simulink model "autoquet_simulink"  (R2023b)
settings: Solver=FixedStepAuto  StartTime=0.0  StopTime=600  FixedStep=1e-3  RelTol=1e-3
libraries: arduinolib x8, dspfdesign x2, arduinosensorlib x1
settings Model: ExtModeTrigDuration=2  Creator=doria  LastModifiedBy=doria
settings OptimizationCC: EnhancedBackFolding=on  PassReuseOutputArgsAs=Individual arguments  ZeroExternalMemoryAtStartup=off  ZeroInternalMemoryAtStartup=off  MaxStackSize=64  OptimizeBlockOrder=speed  DifferentSizesBufferReuse=on  OptimizationCustomize=off  EfficientTunableParamExpr=on
settings DebuggingCC: ParameterTunabilityLossMsg=error
settings HardwareCC: ProdBitPerInt=16  ProdBitPerPointer=16  ProdBitPerSizeT=16  ProdBitPerPtrDiffT=16  ProdLargestAtomicFloat=None  ProdWordSize=8  ProdHWDeviceType=Atmel->AVR
settings SFSimCC: MATLABDynamicMemAlloc=off
settings RTWCC: Description=Embedded Coder  SystemTargetFile=ert.tlc  HardwareBoard=Arduino Leonardo  TemplateMakefile=ert_default_tmf  Toolchain=Arduino AVR  BuildConfiguration=Faster Runs
settings CodeAppCC: ForceParamTrailComments=on  IgnoreCustomStorageClasses=off  OperatorAnnotations=on  SimulinkDataObjDesc=on  SFDataObjDesc=on  InsertBlockDesc=on
settings ERTTargetCC: SupportContinuousTime=on  SupportVariableSizeSignals=on  ExtModeTransport=3  ExtModeStaticAlloc=on  ExtModeAutomaticAllocSize=off  ExtModeStaticAllocSize=250  ExtModeMexFile=ext_xcp  ExtModeIntrfLevel=Level2 - Open

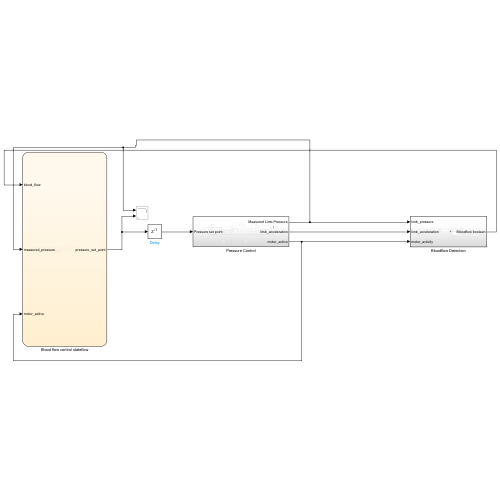
[thumbnail: Simulink's stored preview of the top-level diagram]
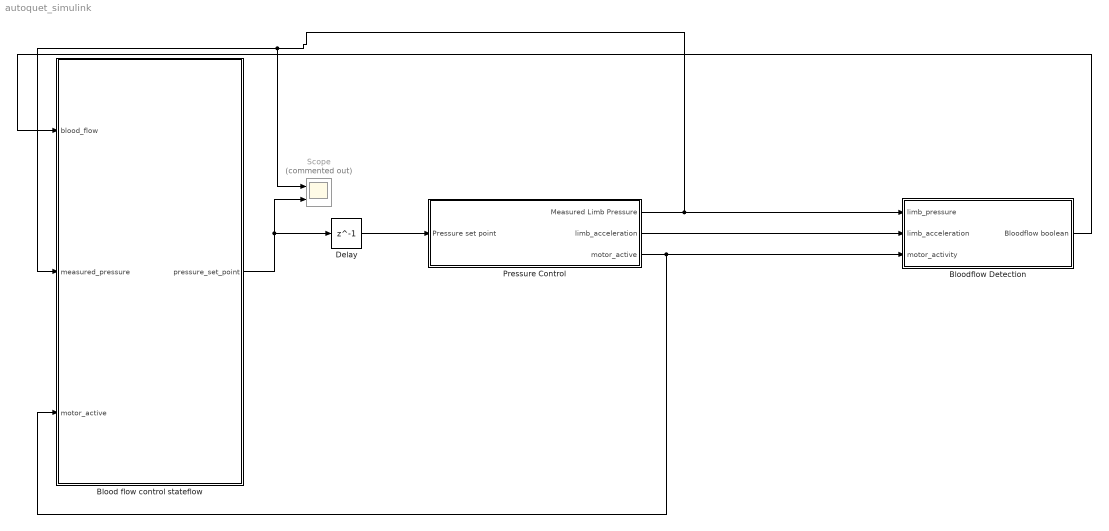
== system autoquet_simulink ==
  Blood flow control stateflow : Stateflow chart  TreatAsAtomicUnit=on
  Bloodflow Detection : Subsystem
  Delay : Delay  DelayLength=1  InitialCondition=100
  Pressure Control : Subsystem
  Scope : Scope  Commented=on  NumInputPorts=2
  wires:
  Delay/1 -> Pressure Control/1(Pressure set point)
  Pressure Control/1(Measured Limb Pressure) -> Bloodflow Detection/1(limb_pressure), Blood flow control stateflow/2(measured_pressure), Scope/1
  Bloodflow Detection/1(Bloodflow boolean) -> Blood flow control stateflow/1(blood_flow)
  Pressure Control/3(motor_active) -> Blood flow control stateflow/3(motor_active), Bloodflow Detection/3(motor_activity)
  Blood flow control stateflow/1(pressure_set_point) -> Delay/1, Scope/2
  Pressure Control/2(limb_acceleration) -> Bloodflow Detection/2(limb_acceleration)

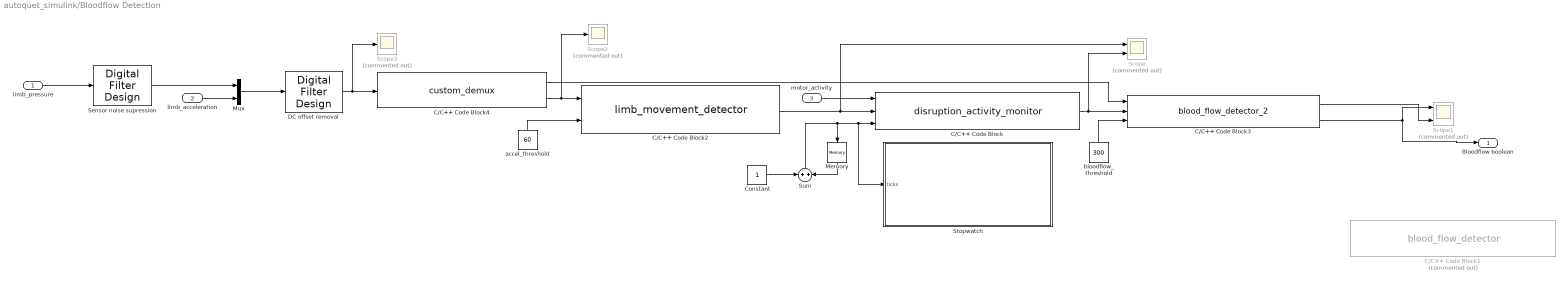
== system autoquet_simulink/Bloodflow Detection ==
  limb_pressure : Inport
  limb_acceleration : Inport  Port=2
  motor_activity : Inport  Port=3
  C/C++ Code Block : S-Function  FunctionName=disruption_activity_monitor  SFunctionModules=disruption_activity_monitor_wrapper.c  SFunctionDeploymentMode=off  EnableBusSupport=off  mask(S-Function Builder){}
      mask help: Simulink:masks:SFunctionBuilder_MD
      mask init:
      | val = [[.9  0.75 0.75 1 1 .9 .9 1]',[1 1 0.75 0.75 .9 .9 1 .9]'];try , sys = get_param(gcb,'SfunBuilderFcnName');if isempty(sys), sys = get_param(gcb,'FunctionName'); end,catch, sys = get_param(gcb,'FunctionName'); end
      settings: CopyFcn=set_param(gcbh,'LinkStatus','none')  OpenFcn=sfunctionwizard(gcbh)
      mask Display:
      | plot(val(:,1),val(:,2))
      | disp(sys)
      | port_label('input',1,'motor_active')
      | port_label('input',2,'movement_detected')
      | port_label('input',3,'time')
      | port_label('output',1,'pause_summation')
  C/C++ Code Block1 : S-Function  Commented=on  FunctionName=blood_flow_detector  SFunctionModules=blood_flow_detector_wrapper.c  SFunctionDeploymentMode=off  EnableBusSupport=off  mask(S-Function Builder){}
      mask help: Simulink:masks:SFunctionBuilder_MD
      mask init: same as autoquet_simulink/Bloodflow Detection/C/C++ Code Block
      settings: CopyFcn=set_param(gcbh,'LinkStatus','none')  OpenFcn=sfunctionwizard(gcbh)
      mask Display: plot(val(:,1),val(:,2)),disp(sys),port_label('input',1,'u0'),port_label('input',2,'disruption_active'),port_label('input',3,'bloodflow_threshold'),port_label('output',1,'y0'),port_label('output',2,'bloodflow_boolean')
  C/C++ Code Block2 : S-Function  FunctionName=limb_movement_detector  SFunctionModules=limb_movement_detector_wrapper.c  SFunctionDeploymentMode=off  EnableBusSupport=off  mask(S-Function Builder){}
      mask help: Simulink:masks:SFunctionBuilder_MD
      mask init: same as autoquet_simulink/Bloodflow Detection/C/C++ Code Block
      settings: CopyFcn=set_param(gcbh,'LinkStatus','none')  OpenFcn=sfunctionwizard(gcbh)
      mask Display:
      | plot(val(:,1),val(:,2))
      | disp(sys)
      | port_label('input',1,'limb_acceleration')
      | port_label('input',2,'accel_threshold')
      | port_label('output',1,'movement_boolean')
  C/C++ Code Block3 : S-Function  FunctionName=blood_flow_detector_2  SFunctionModules=blood_flow_detector_2_wrapper.c  SFunctionDeploymentMode=off  EnableBusSupport=off  mask(S-Function Builder){}
      mask help: Simulink:masks:SFunctionBuilder_MD
      mask init: same as autoquet_simulink/Bloodflow Detection/C/C++ Code Block
      settings: CopyFcn=set_param(gcbh,'LinkStatus','none')  OpenFcn=sfunctionwizard(gcbh)
      mask Display:
      | plot(val(:,1),val(:,2))
      | disp(sys)
      | port_label('input',1,'u0')
      | port_label('input',2,'disruption_active')
      | port_label('input',3,'bloodflow_threshold')
      | port_label('output',1,'y0')
      | port_label('output',2,'bloodflow_boolean')
  C/C++ Code Block4 : S-Function  FunctionName=custom_demux  SFunctionModules=custom_demux_wrapper.c  SFunctionDeploymentMode=off  EnableBusSupport=off  mask(S-Function Builder){}
      mask help: Simulink:masks:SFunctionBuilder_MD
      mask init: same as autoquet_simulink/Bloodflow Detection/C/C++ Code Block
      settings: CopyFcn=set_param(gcbh,'LinkStatus','none')  OpenFcn=sfunctionwizard(gcbh)
      mask Display:
      | plot(val(:,1),val(:,2))
      | disp(sys)
      | port_label('input',1,'combined_vector')
      | port_label('output',1,'filtered_pressure')
      | port_label('output',2,'filtered_acceleration')
  Constant : Constant  OutDataTypeStr=uint32  SampleTime=0.1
  DC offset removal : dspfdesign/Digital Filter Design  mwdsp_browser_bugfix_var=off
  Memory : Memory
  Mux : Mux  Inputs=2
  Scope : Scope  Commented=on  NumInputPorts=2
  Scope1 : Scope  Commented=on  NumInputPorts=2
  Scope2 : Scope  Commented=on
  Scope3 : Scope  Commented=on
  Sensor noise supression : dspfdesign/Digital Filter Design  mwdsp_browser_bugfix_var=off
  Stopwatch : Subsystem
  Sum : Sum  Inputs=+|+
  accel_threshold : Constant  Value=60  OutDataTypeStr=uint16
  bloodflow_threshold : Constant  Value=300  OutDataTypeStr=uint16
  Bloodflow boolean : Outport
  wires:
  Mux/1 -> DC offset removal/1
  C/C++ Code Block/1 -> C/C++ Code Block3/2, Scope/2
  motor_activity/1 -> C/C++ Code Block/1
  C/C++ Code Block3/2 -> Bloodflow boolean/1, Scope1/1
  bloodflow_threshold/1 -> C/C++ Code Block3/3
  C/C++ Code Block3/1 -> Scope1/2
  Constant/1 -> Sum/1
  Memory/1 -> Sum/2
  accel_threshold/1 -> C/C++ Code Block2/2
  limb_pressure/1 -> Sensor noise supression/1
  Sensor noise supression/1 -> Mux/1
  DC offset removal/1 -> Scope3/1, C/C++ Code Block4/1
  C/C++ Code Block2/1 -> Scope/1, C/C++ Code Block/2
  Sum/1 -> Stopwatch/1(ticks), C/C++ Code Block/3, Memory/1
  limb_acceleration/1 -> Mux/2
  C/C++ Code Block4/1 -> C/C++ Code Block3/1
  C/C++ Code Block4/2 -> Scope2/1, C/C++ Code Block2/1

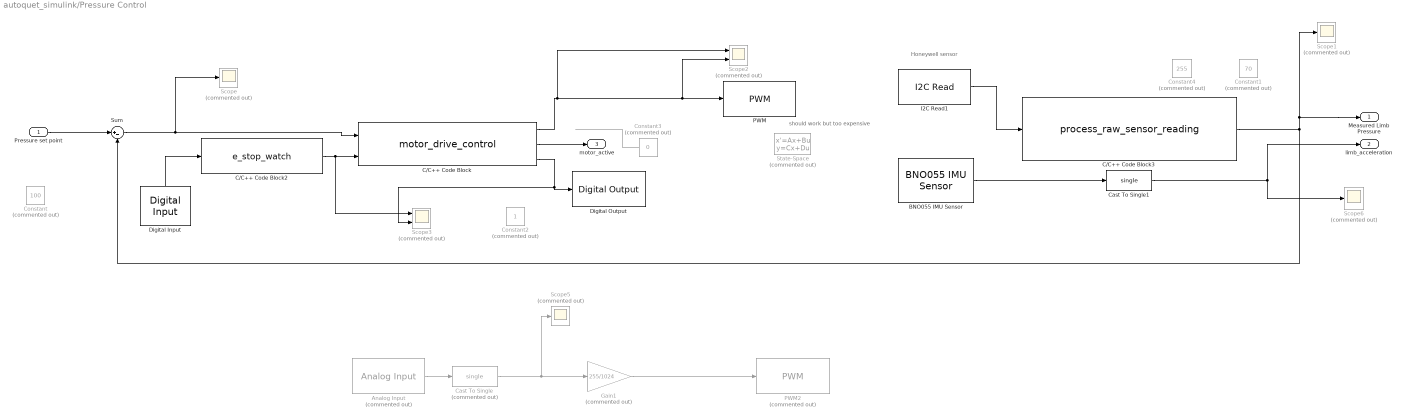
== system autoquet_simulink/Pressure Control ==
  note: should work but too expensive
  note: Honeywell sensor
  Pressure set point : Inport
  Analog Input : arduinolib/Analog Input  Commented=on  pinNumber=0  ReadResultsOnly=off  ConversionTriggerSource=Software  ExternalTriggerType=uint32( 0 )  OutputDataType=uint16  EnableConversionCompleteNotify=off  EnableOuputStatus=off  SampleTime=-1  blockPlatform=arduino
  BNO055 IMU Sensor : arduinosensorlib/BNO055 IMU Sensor  SlaveAddress=0x29  OperationMode=Fusion  Accel=on  AngularRate=off  MagField=off  EulerAngles=off  Quat=off  LinearAccel=off  GravityVector=off  Status=off  Timestamp=off  AccelRange=4G  AccelBW=62.5 Hz  GyroRange=2000 dps  GyroBW=32 Hz  MagODR=10 Hz  spf=1  SampleTime=0.1  blockPlatform=ARDUINO  QueueSizeFactor=1
  C/C++ Code Block : S-Function  FunctionName=motor_drive_control  SFunctionModules=motor_drive_control_wrapper.c  SFunctionDeploymentMode=off  EnableBusSupport=off  mask(S-Function Builder){}
      mask help: Simulink:masks:SFunctionBuilder_MD
      mask init: same as autoquet_simulink/Bloodflow Detection/C/C++ Code Block
      settings: CopyFcn=set_param(gcbh,'LinkStatus','none')  OpenFcn=sfunctionwizard(gcbh)
      mask Display:
      | plot(val(:,1),val(:,2))
      | disp(sys)
      | port_label('input',1,'limb_pressure_diff')
      | port_label('input',2,'emergency_stop')
      | port_label('output',1,'inflation_state')
      | port_label('output',2,'motor_active')
      | port_label('output',3,'solenoid_state')
  C/C++ Code Block2 : S-Function  FunctionName=e_stop_watch  SFunctionModules=e_stop_watch_wrapper.c  SFunctionDeploymentMode=off  EnableBusSupport=off  mask(S-Function Builder){}
      mask help: Simulink:masks:SFunctionBuilder_MD
      mask init: same as autoquet_simulink/Bloodflow Detection/C/C++ Code Block
      settings: CopyFcn=set_param(gcbh,'LinkStatus','none')  OpenFcn=sfunctionwizard(gcbh)
      mask Display:
      | plot(val(:,1),val(:,2))
      | disp(sys)
      | port_label('input',1,'arduino_input')
      | port_label('output',1,'estop')
  C/C++ Code Block3 : S-Function  FunctionName=process_raw_sensor_reading  SFunctionModules=process_raw_sensor_reading_wrapper.c  SFunctionDeploymentMode=off  EnableBusSupport=off  mask(S-Function Builder){}
      mask help: Simulink:masks:SFunctionBuilder_MD
      mask init: same as autoquet_simulink/Bloodflow Detection/C/C++ Code Block
      settings: CopyFcn=set_param(gcbh,'LinkStatus','none')  OpenFcn=sfunctionwizard(gcbh)
      mask Display:
      | plot(val(:,1),val(:,2))
      | disp(sys)
      | port_label('input',1,'raw_sensor_input')
      | port_label('output',1,'limb_pressure_mmhg')
  Cast To Single : DataTypeConversion  Commented=on  OutDataTypeStr=single  SaturateOnIntegerOverflow=off  RndMeth=Floor
  Cast To Single1 : DataTypeConversion  OutDataTypeStr=single  SaturateOnIntegerOverflow=off  RndMeth=Floor
  Constant : Constant  Commented=on  Value=100  OutDataTypeStr=single  SampleTime=0.1
  Constant1 : Constant  Commented=on  Value=70  OutDataTypeStr=single
  Constant2 : Constant  Commented=on  OutDataTypeStr=boolean
  Constant3 : Constant  Commented=on  Value=0  OutDataTypeStr=boolean
  Constant4 : Constant  Commented=on  Value=255  OutDataTypeStr=single
  Digital Input : arduinolib/Digital Input  pinNumber=0  mode=Default  Direction=input  SampleTime=0.1  blockPlatform=arduino
  Digital Output : arduinolib/Digital Output  pinNumber=10  Direction=output  blockPlatform=arduino
  Gain1 : Gain  Commented=on  Gain=255/1024  ParamDataTypeStr=single
  I2C Read1 : arduinolib/I2C Read  I2CModule=0  Mode=Master  SlaveAddress=0x28  SlaveByteOrder=BigEndian  Direction=Receiver  RegisterAddressMode=off  RegisterAddress=1  SlaveDataType=uint8  DataLength=2  NoAck=off  RepeatedStart=off  OutputStatus=off  blockPlatform=ARDUINO  SampleTime=0.1
  PWM : arduinolib/PWM  pinNumber=5  frequencyType=Default  desiredFrequency=490.2  achievableFrequency=490.2
  PWM2 : arduinolib/PWM  Commented=on  pinNumber=3  frequencyType=Default  desiredFrequency=490.2  achievableFrequency=490.2
  Scope{,1,5..6} (4 alike) : Scope  Commented=on
  Scope2 : Scope  Commented=on  NumInputPorts=2
  Scope3 : Scope  Commented=on  NumInputPorts=2
  State-Space : StateSpace  Commented=on  A=-1  D=0  InitialCondition=255
  Sum : Sum  Inputs=|+-
  Measured Limb Pressure : Outport
  limb_acceleration : Outport  Port=2
  motor_active : Outport  Port=3
  wires:
  Analog Input/1 -> Cast To Single/1
  Gain1/1 -> PWM2/1
  C/C++ Code Block3/1 -> Scope1/1, Measured Limb Pressure/1, Sum/2
  Cast To Single/1 -> Scope5/1, Gain1/1
  Digital Input/1 -> C/C++ Code Block2/1
  C/C++ Code Block2/1 -> Scope3/1, C/C++ Code Block/2
  C/C++ Code Block/2 -> motor_active/1
  C/C++ Code Block/3 -> Scope3/2, Digital Output/1
  I2C Read1/1 -> C/C++ Code Block3/1
  BNO055 IMU Sensor/1 -> Cast To Single1/1
  Cast To Single1/1 -> Scope6/1, limb_acceleration/1
  Sum/1 -> Scope/1, C/C++ Code Block/1
  Constant3/1 -> ?
  C/C++ Code Block/1 -> Scope2/2, PWM/1, Scope2/1
  Pressure set point/1 -> Sum/1

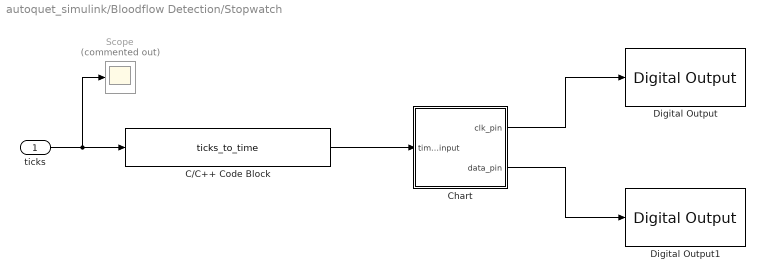
== system autoquet_simulink/Bloodflow Detection/Stopwatch ==
  ticks : Inport
  C/C++ Code Block : S-Function  FunctionName=ticks_to_time  SFunctionModules=ticks_to_time_wrapper.c  SFunctionDeploymentMode=off  EnableBusSupport=off  mask(S-Function Builder){}
      mask help: Simulink:masks:SFunctionBuilder_MD
      mask init: same as autoquet_simulink/Bloodflow Detection/C/C++ Code Block
      settings: CopyFcn=set_param(gcbh,'LinkStatus','none')  OpenFcn=sfunctionwizard(gcbh)
      mask Display:
      | plot(val(:,1),val(:,2))
      | disp(sys)
      | port_label('input',1,'ticks_elapsed')
      | port_label('output',1,'binary_time')
  Chart : Stateflow chart  TreatAsAtomicUnit=on
  Digital Output : arduinolib/Digital Output  pinNumber=8  Direction=output  blockPlatform=arduino
  Digital Output1 : arduinolib/Digital Output  pinNumber=9  Direction=output  blockPlatform=arduino
  Scope : Scope  Commented=on
  wires:
  Chart/1(clk_pin) -> Digital Output/1
  Chart/2(data_pin) -> Digital Output1/1
  C/C++ Code Block/1 -> Chart/1(time_input)
  ticks/1 -> Scope/1, C/C++ Code Block/1

== stateflow chart autoquet_simulink/Bloodflow Detection/Stopwatch/Chart ==
  state send_data
    exit:
    clk_pin = true
    word_iterator = 1
    state data_high
      entry:
      data_pin = true
    state ack_bit
      entry:
      clk_pin = false
      exit:
      data_pin = false
      clk_pin = true
    state latch_data
      entry:
      clk_pin = true
      buffer = bitshift(buffer, -1)
      bit_iterator = bit_iterator + 1
    state buffer_reset
      entry:
      buffer = time_input(word_iterator-1)
      exit:
      bit_iterator = 1
    state reset_clk
      entry:
      clk_pin = false
    state post_ack_reset
      entry:
      word_iterator = word_iterator + 1
    state idler
      exit:
      clk_pin = false
    state data_low
      entry:
      data_pin = false
    reset_clk -> data_high [order 2] : [bitand(buffer, 1) == 1]
    data_high -> latch_data
    (default) -> reset_clk
    post_ack_reset -> buffer_reset : [word_iterator <= len]
    latch_data -> ack_bit [order 2] : [bit_iterator > 8]
    latch_data -> reset_clk [order 1] : [bit_iterator <= 8]
    buffer_reset -> reset_clk
    reset_clk -> data_low [order 1] : [bitand(buffer, 1) == 0]
    idler -> post_ack_reset
    data_low -> latch_data
    ack_bit -> idler
  state Start_signal
    entry:
    data_pin = false
    buffer = command
    bit_iterator = 1
    word_iterator = 1
  state Stop
    entry:
    transmit = false
    exit:
    data_pin = true
  state init
    entry:
    command_state = 0
    transmit = false
    data_pin = true
    clk_pin = true
  state command_flow
    state find_command
    state transmit_data
      entry:
      command = 192
      len = 5
      command_state = command_state + 1
      transmit = true
    state data_directive
      entry:
      command = 64
      len = 1
      command_state = command_state + 1
      transmit = true
    state display_control
      entry:
      command = 143
      len = 1
      command_state = 0
      transmit = true
    (default) -> find_command
    find_command -> data_directive [order 1] : [command_state == 0]
    find_command -> transmit_data [order 2] : [command_state == 1]
    find_command -> display_control [order 3] : [command_state == 2]
  Start_signal -> send_data
  send_data -> Stop : [word_iterator >len]
  Stop -> command_flow
  command_flow -> Start_signal : [transmit == true]
  (default) -> init
  init -> command_flow
  data: clk_pin output; data_pin output boolean; bit_iterator local uint8; buffer local uint8; len local uint8; word_iterator local uint8; time_input input uint8 size=[4,1]; command_state local uint8; transmit local boolean; command local uint8

== stateflow chart autoquet_simulink/Blood flow control stateflow ==
  settings: updateMethod=DISCRETE  sampleTime=0.1
  state Binary_search_ideal_pressure
    % Find ideal pressure to stop bleeding between pressure extremes measured in previous stage
    entry:
    %binary_search_upper = 290 %pressure_upper_bound
    %binary_search_lower = 100 %pressure_lower_bound
    binary_search_upper = pressure_upper_bound
    binary_search_lower = pressure_lower_bound
    ideal_pressure_found = false
    state Too_tight
      entry:
      binary_search_upper = pressure_set_point
    state Adjust_pressure_set_point
      entry:
      pressure_set_point = (binary_search_upper + binary_search_lower)/2
      pressure_difference = binary_search_upper - binary_search_lower
    state Ideal_pressure_found
      entry:
      pressure_set_point = binary_search_upper
      ideal_pressure_found = true
    state Idle
    state Too_loose
      entry:
      binary_search_lower = pressure_set_point
    Too_tight -> Adjust_pressure_set_point
    (junction 112) -> Too_tight [order 3] : [pressure_difference >= 30 ...
        |  && blood_flow == 0]
    (default) -> Adjust_pressure_set_point
    (junction 112) -> Ideal_pressure_found [order 1] : [pressure_difference < 30]
    Binary_search_ideal_pressure.Idle -> (junction 112) : [duration(motor_active == 0) > 5]
    Adjust_pressure_set_point -> Binary_search_ideal_pressure.Idle : [(measured_pressure >= pressure_set_point - 30/2) ...
        | && (measured_pressure  <= pressure_set_point + 30/2)]
    (junction 112) -> Too_loose [order 2] : [pressure_difference >= 30 ...
        |  && blood_flow > 0]
    Too_loose -> Adjust_pressure_set_point
  state Find_initial_bounds
    entry:
    pressure_set_point = 100
    upper_bound_found = false
    state Inflate
      %Inflate quickly to stop blood flow
      exit:
      pressure_upper_bound = pressure_set_point
      state Initial_wait
        % Used to wait out the
        % initial to ensure all
        % data signals are acccurate
        %entry:
        %initial_inflation = true
        %exit:
        %initial_inflation = false
      state Idle
      state Increase_pressure_set_point
        entry:
        pressure_set_point = pressure_set_point + 30 %bulk_increment
      state wait
      (default) -> Initial_wait
      Find_initial_bounds.Inflate.Idle -> Increase_pressure_set_point : [duration(motor_active == 0) > 10]
      wait -> Find_initial_bounds.Inflate.Idle : [measured_pressure >= pressure_set_point]
      Increase_pressure_set_point -> wait
      Initial_wait -> wait : after(1.5,sec)
    state Deflate
      % Slowly deflate until blood flow returns
      exit:
      pressure_lower_bound = pressure_set_point
      state Idle
      state Decrease_pressure_set_point
        entry:
        pressure_set_point = pressure_set_point - 30 %bulk_decrement
      state Wait
      (default) -> Decrease_pressure_set_point
      Wait -> Find_initial_bounds.Deflate.Idle : [measured_pressure<=pressure_set_point]
      Find_initial_bounds.Deflate.Idle -> Decrease_pressure_set_point : [duration(motor_active == 0) > 10]
      Decrease_pressure_set_point -> Wait
    note: 1.5 seconds is for the transport delay
    (default) -> Inflate
    Inflate -> Deflate : [duration(blood_flow == 0) > 5]{upper_bound_found = true}
  state Fine_adjustments [commented out]
    state Increase_pressure [commented out]
      entry:
      pressure_set_point = pressure_set_point + 10 %fine_increment
    state idle [commented out]
    state Default_state [commented out]
    state Decrease_pressure [commented out]
      entry:
      pressure_set_point = pressure_set_point - 10 %fine_decrement
    Default_state -> Increase_pressure [commented out] : [duration(blood_flow>0) > 5]
    (default) -> Default_state [commented out]
    Increase_pressure -> idle [commented out]
    idle -> Default_state [commented out] : [duration(motor_active == 0) > 10]
    Decrease_pressure -> idle [commented out]
    Default_state -> Decrease_pressure [commented out] : [duration(blood_flow ==0) > 5]
  state Idle [commented out]
    % Wait in the idle state for a given amount of time
  (default) -> Binary_search_ideal_pressure [commented out]
  (default) -> Find_initial_bounds
  Fine_adjustments -> Idle [commented out] : [duration(blood_flow == 0) > 10 && [duration(motor_active == 0) > 10]]
  Binary_search_ideal_pressure -> Idle [commented out] : [ideal_pressure_found==true]
  Find_initial_bounds -> Binary_search_ideal_pressure : [(duration(blood_flow>0) > 4) && upper_bound_found == true]
  Idle -> Fine_adjustments [commented out] : [duration(blood_flow > 0) > 10]
  data: pressure_set_point output single; blood_flow input; measured_pressure input single; binary_search_lower local single; binary_search_upper local single; ideal_pressure_found local boolean; pressure_difference local single; pressure_lower_bound local single; pressure_upper_bound local single; upper_bound_found local boolean; motor_active input boolean
